simulink model "untitled1"  (R2022b)
settings: Solver=VariableStepAuto  StartTime=0.0  StopTime=10.0  RelTol=1e-3
settings Model: Creator=hollis  LastModifiedBy=hollis
settings OptimizationCC: DefaultParameterBehavior=Inlined  EnhancedBackFolding=on  PassReuseOutputArgsAs=Individual arguments  ZeroExternalMemoryAtStartup=off  ZeroInternalMemoryAtStartup=off  OptimizeBlockOrder=speed  DifferentSizesBufferReuse=on  OptimizationCustomize=off  EfficientTunableParamExpr=on
settings DebuggingCC: ParameterTunabilityLossMsg=error
settings SFSimCC: MATLABDynamicMemAlloc=off
settings RTWCC: Description=Embedded Coder  SystemTargetFile=ert.tlc  TemplateMakefile=ert_default_tmf
settings CodeAppCC: ForceParamTrailComments=on  IgnoreCustomStorageClasses=off  OperatorAnnotations=on  SimulinkDataObjDesc=on  SFDataObjDesc=on  InsertBlockDesc=on
settings ERTTargetCC: TargetLangStandard=C99 (ISO)  GenerateSampleERTMain=on  InlinedParameterPlacement=NonHierarchical  ERTCustomFileTemplate=example_file_process.tlc

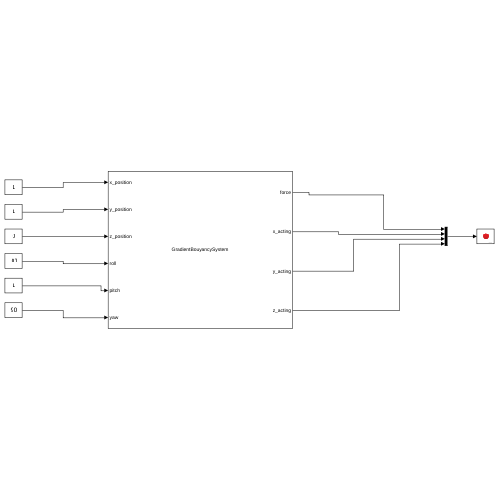
[thumbnail: Simulink's stored preview of the top-level diagram]
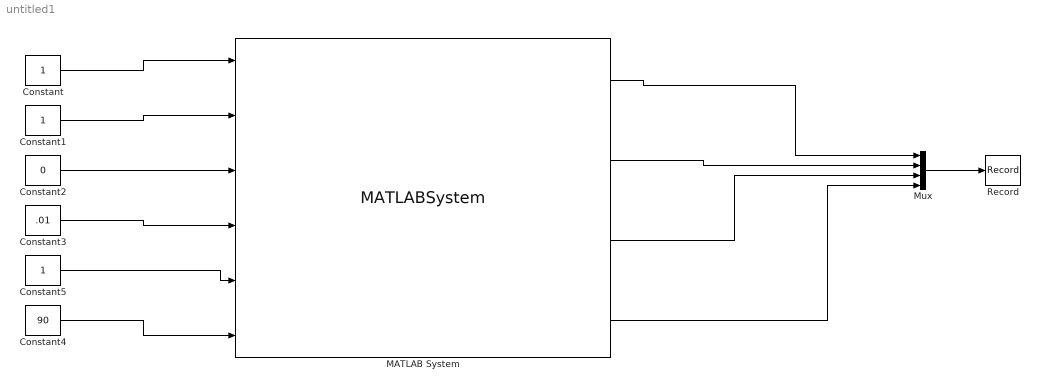
== system untitled1 ==
  Constant : Constant
  Constant1 : Constant
  Constant2 : Constant  Value=0
  Constant3 : Constant  Value=.01
  Constant4 : Constant  Value=90
  Constant5 : Constant
  MATLAB System : MATLABSystem  System=GradientBouyancySystem  SimulateUsing=Interpreted execution
      mask Type: GradientBouyancySystem
      mask Display:
      | disp('GradientBouyancySystem');
      | port_label('input',1,'x_position');
      | port_label('input',2,'y_position');
      | port_label('input',3,'z_position');
      | port_label('input',4,'roll');
      | port_label('input',5,'pitch');
      | port_label('input',6,'yaw');
      | port_label('output',1,'force');
      | port_label('output',2,'x_acting');
      | port_label('output',3,'y_acting');
      | port_label('output',4,'z_acting');
  Mux : Mux
  Record : Record  FileSettingsInternal="{\"entries\":[{\"content\":{\"excelSettings\":{\"content\":{},\"type\":\"Streamout.ExcelSettings\"}},\"type\":\"Streamout.FileSettingStorage\",\"uuid\":\"62d5ee9c-08ef-4726-9b58-1e61b88580f4\"}],\"packageUris\":[\"http://schema.mathworks.com/mf0/streamout_blocks/R2020a\"],\"version\":\"1.0\"}"  SignalsInternal="{\"entries\":[{\"content\":{\"signals\":[{\"content\":{\"blockPath\":[\"untitled1/Record\"],\"channel\":[],\"dimensions\":[4],\"domain\":\"untitled1/Record\",\"hasChildren\":true,\"lineColor\":\"#edb120\",\"plots\":[],\"port\":1,\"sid\":[\"\"],\"signalID\":255,\"signalName\":\"Mux\"},\"type\":\"RecordBlkView.Signal\",\"uuid\":\"720c16b3-a769-4fa3-80f8-ef9aea2c1bdf\"},{\"content\":{\"blockPath\":[\"untitled1/Record\"],\"channel\":[1],\"dimensions\":[4],\"domain\":\"untitled1/Record\",\"lineColor\":\"#d95319\",\"parentID\":255,\"plots\":[1],\"port\":1,\"sid\":[\"\"],\"signalID\":256,\"signalName\":\"Mux\"},\"type\":\"RecordBlkView.Signal\",\"uuid\":\"98b81f1e-b1af-43f9-921b-82af96311574\"},{\"content\":{\"blockPath\":[\"untitled1/Record\"],\"channel\":[2],\"dimensions\":[4],\"domain\":\"untitled1/Record\",\"lineColor\":\"#77ac30\",\"parentID\":255,\"plots\":[1],\"port\":1,\"sid\":[\"\"],\"signalID\":260,\"signalName\":\"Mux\"},\"type\":\"RecordBlkView.Signal\",\"uuid\":\"35145e24-45b8-462b-ab97-19c5b2dfdce0\"},{\"content\":{\"blockPath\":[\"untitled1/Record\"],\"channel\":[3],\"dimensions\":[4],\"domain\":\"untitled1/Record\",\"lineColor\":\"#4dbeee\",\"parentID\":255,\"plots\":[1],\"port\":1,\"sid\":[\"\"],\"signalID\":261,\"signalName\":\"Mux\"},\"type\":\"RecordBlkView.Signal\",\"uuid\":\"0fd7f14a-f325-4980-b4c6-8c81c4c39a04\"},{\"content\":{\"blockPath\":[\"untitled1/Record\"],\"channel\":[4],\"dimensions\":[4],\"domain\":\"untitled1/Record\",\"lineColor\":\"#a2142f\",\"parentID\":255,\"plots\":[1],\"port\":1,\"sid\":[\"\"],\"signalID\":262,\"signalName\":\"Mux\"},\"type\":\"RecordBlkView.Signal\",\"uuid\":\"f7a8ae97-1cf3-4201-8226-0352706e5bcb\"}]},\"type\":\"RecordBlkView.InputSignals\",\"uuid\":\"32fa6d65-d834-480b-bcb7-c1a00512d724\"}],\"packageUris\":[\"http://schema.mathworks.com/mf0/streamout_blocks/R2020a\"],\"version\":\"1.0\"}"  VisualizationBindings="{\"sparklinesplugin\":{\"info\":[{\"bindingParametersList\":[],\"subplotID\":1}]}}"
  wires:
  Constant/1 -> MATLAB System/1
  Constant1/1 -> MATLAB System/2
  Constant2/1 -> MATLAB System/3
  Constant4/1 -> MATLAB System/6
  Constant5/1 -> MATLAB System/5
  MATLAB System/1 -> Mux/1
  MATLAB System/2 -> Mux/2
  MATLAB System/3 -> Mux/3
  MATLAB System/4 -> Mux/4
  Mux/1 -> Record/1
  Constant3/1 -> MATLAB System/4
